simulink model "enable_test1"  (R2014a)
settings: Solver=ode45  StartTime=0.0  StopTime=10.0  RelTol=1e-3
settings Model: CovSFcnEnable=on  Creator=hamza  LastModifiedBy=hbourbou
settings DataIOCC: LimitDataPoints=off  SaveFormat=StructureWithTime
settings DebuggingCC: MergeDetectMultiDrivingBlocksExec=error  SolverPrmCheckMsg=none  FrameProcessingCompatibilityMsg=error
settings HardwareCC: ProdBitPerPointer=64  ProdLargestAtomicFloat=Float  ProdIntDivRoundTo=Zero  ProdEndianess=LittleEndian  ProdHWDeviceType=Specified
settings ModelReferenceCC: PropagateSignalLabelsOutOfModel=on

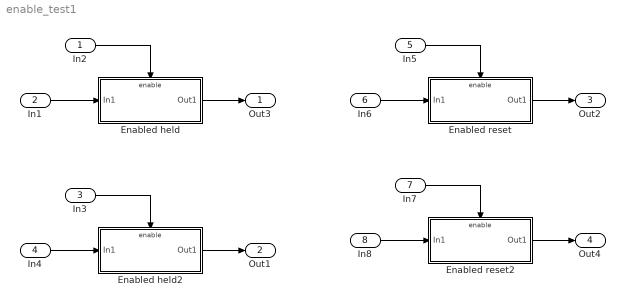
== system enable_test1 ==
  In2 : Inport  OutDataTypeStr=boolean
  In1 : Inport  Port=2
  In3 : Inport  Port=3  OutDataTypeStr=boolean
  In4 : Inport  Port=4  PortDimensions=2
  In5 : Inport  Port=5  OutDataTypeStr=boolean
  In6 : Inport  Port=6
  In7 : Inport  Port=7  OutDataTypeStr=int32
  In8 : Inport  Port=8  PortDimensions=2
  Enabled held : Subsystem  TreatAsAtomicUnit=on
  Enabled held2 : Subsystem  TreatAsAtomicUnit=on
  Enabled reset : Subsystem  TreatAsAtomicUnit=on
  Enabled reset2 : Subsystem  TreatAsAtomicUnit=on
  Out3 : Outport
  Out1 : Outport  Port=2
  Out2 : Outport  Port=3
  Out4 : Outport  Port=4
  wires:
  In2/1 -> Enabled held/Enable
  In1/1 -> Enabled held/1(In1)
  Enabled held/1(Out1) -> Out3/1
  In3/1 -> Enabled held2/Enable
  In4/1 -> Enabled held2/1(In1)
  Enabled held2/1(Out1) -> Out1/1
  In5/1 -> Enabled reset/Enable
  In6/1 -> Enabled reset/1(In1)
  Enabled reset/1(Out1) -> Out2/1
  In7/1 -> Enabled reset2/Enable
  In8/1 -> Enabled reset2/1(In1)
  Enabled reset2/1(Out1) -> Out4/1

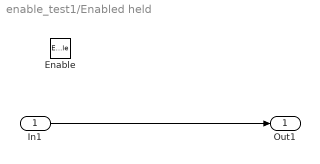
== system enable_test1/Enabled held ==
  In1 : Inport
  Enable : EnablePort
  Out1 : Outport
  wires:
  In1/1 -> Out1/1

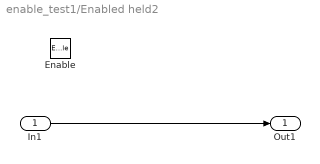
== system enable_test1/Enabled held2 ==
  In1 : Inport
  Enable : EnablePort
  Out1 : Outport
  wires:
  In1/1 -> Out1/1

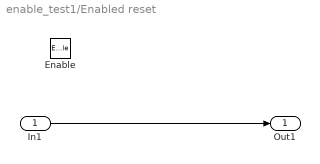
== system enable_test1/Enabled reset ==
  In1 : Inport
  Enable : EnablePort  StatesWhenEnabling=reset
  Out1 : Outport
  wires:
  In1/1 -> Out1/1

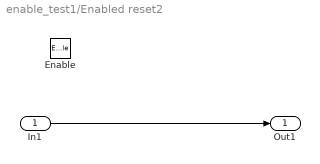
== system enable_test1/Enabled reset2 ==
  In1 : Inport
  Enable : EnablePort  StatesWhenEnabling=reset  ZeroCross=off
  Out1 : Outport
  wires:
  In1/1 -> Out1/1
